simulink model "Three_Phase_Compensated_Network"  (R2021a)
settings: Solver=FixedStepDiscrete  StartTime=0.0  StopTime=0.2  FixedStep=Ts  RelTol=1e-4  EnableMultiTasking=on
PreLoadFcn:
  | Ts=50e-6;
InitFcn:
  | Ts=50e-6;
undefined symbols (not defined in the file or in its folder): D1, Delta, DiscIntNeverNeededParam
libraries: spsSeriesRLCBranchLib x6, spsBreakerLib x6, spsCurrentMeasurementLib x6, spsSurgeArresterLib x6, spsParallelRLCBranchLib x6, spsVoltageMeasurementLib x6, spsThreePhaseSeriesRLCLoadLib x4, spsLoadFlowBusLib x4, spsThreePhaseVIMeasurementLib x3, spsThreePhaseBreakerLib x2, spsDistributedParametersLineLib x2, spsThreePhaseSourceLib x1
(part 1 of 2)
settings Model: ExtModeTrigMode=oneshot  ExtModeArmWhenConnect=off  ExtModeAutoUpdateStatusClock=off  Creator=The MathWorks, Inc.  LastModifiedBy=HP
settings SolverCC: AlgebraicLoopSolver=TrustRegion
settings DataIOCC: SaveFormat=Array  ReturnWorkspaceOutputs=off  SignalLoggingName=sigsOut
settings OptimizationCC: BlockReduction=off  BooleanDataType=off  ExpressionDepthLimit=2147483647  InitFltsAndDblsToZero=on  EfficientMapNaN2IntZero=off  LifeSpan=inf
settings DebuggingCC: UnderspecifiedInitializationDetection=Classic  MergeDetectMultiDrivingBlocksExec=none  CheckExecutionContextPreStartOutputMsg=on  SignalResolutionControl=TryResolveAllWithWarning  MultiTaskDSMMsg=warning  MultiTaskCondExecSysMsg=none  FcnCallInpInsideContextMsg=warning  UnconnectedInputMsg=none  UnconnectedOutputMsg=none  StateNameClashWarn=warning  SFUnexpectedBacktrackingDiag=warning  SFNoUnconditionalDefaultTransitionDiag=warning  SFExecutionAtInitializationDiag=none  SFMachineParentedDataDiag=warning  ArithmeticOperatorsInVariantConditions=warning
settings HardwareCC: ProdBitPerPointer=32  ProdBitPerSizeT=32  ProdBitPerPtrDiffT=32  ProdLargestAtomicFloat=None  ProdIntDivRoundTo=Undefined  ProdEndianess=Unspecified  ProdWordSize=32  ProdHWDeviceType=Specified  TargetUnknown=on
settings ModelReferenceCC: PropagateSignalLabelsOutOfModel=off
settings SFSimCC: SimUseLocalCustomCode=off  CustomCodeUndefinedFunction=UseInterfaceOnly
settings RTWCC: RTWUseLocalCustomCode=off
settings CodeAppCC: StateflowObjectComments=on
settings GRTTargetCC: TargetLangStandard=C89/C90 (ANSI)  CombineOutputUpdateFcns=off  GRTInterface=on
settings ConfigComp: CovMetricSettings=dw  CovSaveCumulativeToWorkspaceVar=on  CovSaveSingleToWorkspaceVar=on  CovExternalEMLEnable=off  CovSFcnEnable=off
settings SimscapeCC: SimscapeNormalizeSystem=off

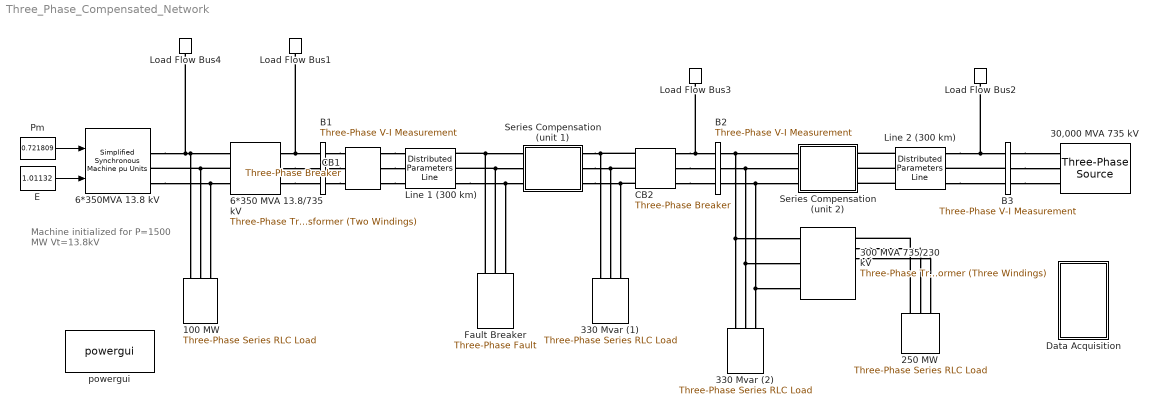
== system Three_Phase_Compensated_Network ==
  note: Machine initialized for
      |  P=1500 MW
      |  Vt=13.8kV
  100 MW : spsThreePhaseSeriesRLCLoadLib/Three-Phase Series RLC Load  LConnTagsString=A|B|C  Configuration=Y (grounded)  NominalVoltage=13.8e3  Vabc=[1e3 1e3 1e3]  Vabcp=[1e3 1e3 1e3]  NominalFrequency=60  UnbalancedPower=off  ActivePower=100000000  InductivePower=0  CapacitivePower=0  Pabc=[10e3 9e3 11e3]  QLabc=[100 90 110]  QCabc=[100 90 110]  Pabcp=[10e3 9e3 11e3]  QLabcp=[100 90 110]  QCabcp=[100 90 110]  Measurements=None  LoadType=constant Z
  250 MW : spsThreePhaseSeriesRLCLoadLib/Three-Phase Series RLC Load  LConnTagsString=A|B|C  Configuration=Y (grounded)  NominalVoltage=230e3  Vabc=[1e3 1e3 1e3]  Vabcp=[1e3 1e3 1e3]  NominalFrequency=60  UnbalancedPower=off  ActivePower=250000000  InductivePower=0  CapacitivePower=0  Pabc=[10e3 9e3 11e3]  QLabc=[100 90 110]  QCabc=[100 90 110]  Pabcp=[10e3 9e3 11e3]  QLabcp=[100 90 110]  QCabcp=[100 90 110]  Measurements=None  LoadType=constant Z
  30,000 MVA 735 kV : spsThreePhaseSourceLib/Three-Phase Source  InternalConnection=Yg  VoltagePhases=off  Voltage=(735000)*0.98865  PhaseAngle=-2.0892  Voltage_phases=[25e3 25e3 25e3]/sqrt(3)  PhaseAngles_phases=[0 -120 +120]  Frequency=60  NonIdealSource=on  SpecifyImpedance=on  Resistance=735^2/30000/10  Inductance=735^2/30000/377  ShortCircuitLevel=30000e6  BaseVoltage=735e3  XRratio=10  BusType=swing  Pref=0  Qref=0  Prefabc=[10e3, 10e3, 10e3]  Qrefabc=[0, 0, 0]  Qmin=-Inf  Qmax=Inf
  300 MVA 735/230 kV : spsThreePhaseTransformerThreeWindingsLib/Three-Phase Transformer (Three Windings)  Winding1Connection=Yg  Winding2Connection=Yg  Winding3Connection=Delta (D1)  CoreType=Three single-phase transformers  SetSaturation=on  Hysteresis=off  DataFile='hysteresis'  SetInitialFlux=off  Measurements=None  UNITS=pu  NominalPower=[ 300e6 , 60 ]  Winding1=[ 735e3 , 0.002 , 0.15 ]  Winding2=[ 230e3 , 0.002 , 0 ]  Winding3=[ 25e3 , 0.05 , 0.20 ]  Rm=500  Lm=1000  L0=0.5  Saturation="[  0,0  ;  0.0012,1.2  ;  1.0,1.45 ]"  InitialFluxes=[-1.02015948080927 0.506449133666723 0.513710347142544]  BreakLoop=on  DiscreteSolver=Trapezoidal iterative  DataType=off  TransfoNumber=0
      settings: AttributesFormatString=\n  SourceProductBaseCode=PS
  330 Mvar (1) : spsThreePhaseSeriesRLCLoadLib/Three-Phase Series RLC Load  LConnTagsString=A|B|C  Configuration=Y (grounded)  NominalVoltage=735e3  Vabc=[1e3 1e3 1e3]  Vabcp=[1e3 1e3 1e3]  NominalFrequency=60  UnbalancedPower=off  ActivePower=1320000  InductivePower=330e6  CapacitivePower=0  Pabc=[10e3 9e3 11e3]  QLabc=[100 90 110]  QCabc=[100 90 110]  Pabcp=[10e3 9e3 11e3]  QLabcp=[100 90 110]  QCabcp=[100 90 110]  Measurements=None  LoadType=constant Z
  "330 Mvar (2) " : spsThreePhaseSeriesRLCLoadLib/Three-Phase Series RLC Load  LConnTagsString=A|B|C  Configuration=Y (grounded)  NominalVoltage=735e3  Vabc=[1e3 1e3 1e3]  Vabcp=[1e3 1e3 1e3]  NominalFrequency=60  UnbalancedPower=off  ActivePower=1320000  InductivePower=330e6  CapacitivePower=0  Pabc=[10e3 9e3 11e3]  QLabc=[100 90 110]  QCabc=[100 90 110]  Pabcp=[10e3 9e3 11e3]  QLabcp=[100 90 110]  QCabcp=[100 90 110]  Measurements=None  LoadType=constant Z
  6*350 MVA 13.8/735 kV : spsThreePhaseTransformerTwoWindingsLib/Three-Phase Transformer (Two Windings)  Winding1Connection=Delta (D1)  Winding2Connection=Yg  CoreType=Three single-phase transformers  SetSaturation=off  Hysteresis=off  DataFile='hysteresis'  SetInitialFlux=off  Measurements=None  UNITS=pu  NominalPower=[ 6*350e6 , 60 ]  Winding1=[ 13.8e3 , 0.002 , 0.08 ]  Winding2=[ 735e3 , 0.002 , 0.08 ]  Rm=500  Lm=500  L0=0.5  Saturation=[ 0,0 ; 0.0024,1.2 ; 1.0,1.52 ]  InitialFluxes=[ 0.8 , -0.8 , 0.7 ]  BreakLoop=off  DiscreteSolver=Trapezoidal iterative  DataType=off  TransfoNumber=0
  6*350MVA 13.8 kV : spsSimplifiedSynchronousMachinepuUnitsLib/Simplified Synchronous Machine pu Units  ConnectionType=3-wire Y  MechanicalLoad=Mechanical power Pm  MeasurementBus=off  NominalParameters="[ 6*350e6 13.8e3  60 ]"  Mechanical=[ inf,0,2 ]  InternalRL="[ 0.22/15  0.22 ]"  InitialConditions=[0 1.43122 0.716215 0.716215 0.716215 -3.34575 -123.346 116.654 ]  IterativeDiscreteModel=Trapezoidal non iterative  TsBlock=-1  TsPowergui=0  LoadFlowParameters=[1,0,0,0,0]  Units=0  BusType=PV  Pref=1500000000  Qref=0  Qmin=-Inf  Qmax=Inf  PLF=0  QLF=0
      settings: AttributesFormatString=\n  SourceProductBaseCode=PS
  B1 : spsThreePhaseVIMeasurementLib/Three-Phase V-I Measurement  VoltageMeasurement=phase-to-ground  SetLabelV=on  LabelV=Vabc_B1  Vpu=on  VpuLL=off  CurrentMeasurement=yes  SetLabelI=on  LabelI=Iabc_B1  Ipu=on  Pbase=100e6  Vbase=735e3  OutputType=Complex  PhasorSimulation=off  PSBequivalent=0
  B2 : spsThreePhaseVIMeasurementLib/Three-Phase V-I Measurement  VoltageMeasurement=phase-to-ground  SetLabelV=on  LabelV=Vabc_B2  Vpu=on  VpuLL=off  CurrentMeasurement=yes  SetLabelI=on  LabelI=Iabc_B2  Ipu=on  Pbase=100e6  Vbase=735e3  OutputType=Complex  PhasorSimulation=off  PSBequivalent=0
  B3 : spsThreePhaseVIMeasurementLib/Three-Phase V-I Measurement  VoltageMeasurement=no  SetLabelV=on  LabelV=Vabc_B3  Vpu=on  VpuLL=off  CurrentMeasurement=no  SetLabelI=on  LabelI=Iabc_B3  Ipu=on  Pbase=100e6  Vbase=735e3  OutputType=Complex  PhasorSimulation=off  PSBequivalent=0
  CB1 : spsThreePhaseBreakerLib/Three-Phase Breaker  InitialState=closed  SwitchA=on  SwitchB=on  SwitchC=on  SwitchTimes="[5/60  ]"  External=off  BreakerResistance=0.001  SnubberResistance=1e5  SnubberCapacitance=inf  Measurements=None
      settings: AttributesFormatString=\n
  CB2 : spsThreePhaseBreakerLib/Three-Phase Breaker  InitialState=closed  SwitchA=on  SwitchB=on  SwitchC=on  SwitchTimes="[5/60  ]"  External=off  BreakerResistance=0.001  SnubberResistance=1e5  SnubberCapacitance=inf  Measurements=None
      settings: AttributesFormatString=\n
  Data Acquisition : Subsystem  mask(Data Acquisition){}
      mask Display: disp('Scopes')
  E : Constant  Value=1.01132
  Fault Breaker : spsThreePhaseFaultLib/Three-Phase Fault  InitialStates=0  FaultA=on  FaultB=off  FaultC=off  GroundFault=on  SwitchTimes=[ 1/60 6/60]  External=off  SwitchStatus=NaN  FaultResistance=0.001  GroundResistance=1  SnubberResistance=inf  SnubberCapacitance=inf  Measurements=Fault currents
  Line 1 (300 km) : spsDistributedParametersLineLib/Distributed Parameters Line  Phases=3  Length=300  Frequency=60  Resistance=[0.01273 0.3864]  Inductance="[0.9337e-3  4.1264e-3]"  Capacitance=[12.74e-9 7.751e-9]  x1=[-0.0017 -7.353032972499e-08 0 0;-0.00165 -7.42667095508993e-08 0 0;-0.0016 -7.49767027685348e-08 0 0;-0.00155 -7.56600571206871e-08 0 0;-0.0015 -7.63165298148087e-08 0 0;-0.00145 -7.69458876092773e-08 0 0;-0.0014 -7.75479068962652e-08 0 0;-0.00135 -7.81223737811864e-08 0 0;-0.0013 -7.86690841586921e-08 0 0;-0.00125 -7.91878437851883e-08 0 0;-0.0012 -7.96784683478498e-08 0 0;-0.00115 -8.01407835301058e-08 0 0;-0.0011 -8.05746250735734e-08 0 0;-0.00105 -8.09798388364179e-08 298982.56569214 -680729.342896262;-0.001 -8.13562808481189e-08 311760.155284904 -674973.083751637;-0.00095 -8.17038173606221e-08 324426.977978977 -668977.009884319;-0.0009 -8.20223248958594e-08 336978.533312573 -662743.251670802;-0.00085 -8.23116902896202e-08 349410.361777845 -656274.023935697;-0.0008 -8.25718107317579e-08 361718.046405336 -649571.625164814;-0.00075 -8.28025938027181e-08 373897.214333303 -642638.436688521;-0.0007 -8.30039575063745e-08 385943.538361373 -635476.921835672;-0.00065 -8.3175830299162e-08 397852.738487979 -628089.625058393;-0.0006 -8.33181511154957e-08 409620.583431022 -620479.171028054;-0.00055 -8.34308693894673e-08 421242.89213123 -612648.263702733;-0.0005 -8.35139450728108e-08 432715.535237661 -604599.685366516;-0.00045 -8.35673486491314e-08 444034.436574848 -596336.29564096;-0.0004 -8.35910611443928e-08 455195.574591042 -587861.030469089;-0.00035 -8.35850741336582e-08 466194.983787052 -579176.901072262;-0.0003 -8.35493897440842e-08 477028.756125164 -570286.992880304;-0.00025 -8.34840206541644e-08 487693.042417654 -561194.464435263;-0.0002 -8.33889900892251e-08 498184.053694381 -551902.546269203;-0.00015 -8.32643318131737e-08 508498.062548993 -542414.539756402;-0.0001 -8.3110090116502e-08 518631.404463254 -532733.815940397;-5e-05 -8.29263198005504e-08 528580.479109035 -522863.814336262]  x2=[-0.0017 -2.16943566485558e-08 0 0;-0.00165 -2.19441858844851e-08 0 0;-0.0016 -2.21862184556595e-08 0 0;-0.00155 -2.24203683690588e-08 0 0;-0.0015 -2.26465524323339e-08 0 0;-0.00145 -2.2864690283364e-08 0 0;-0.0014 -2.30747044188093e-08 0 0;-0.00135 -2.32765202216475e-08 0 0;-0.0013 -2.34700659876849e-08 0 0;-0.00125 -2.36552729510324e-08 0 0;-0.0012 -2.38320753085377e-08 0 0;-0.00115 -2.40004102431651e-08 0 0;-0.0011 -2.4160217946314e-08 0 0;-0.00105 -2.43114416390682e-08 112715.55611075 -734159.055210883;-0.001 -2.44540275923699e-08 126533.2909278 -731904.127817148;-0.00095 -2.45879251461087e-08 140306.069069085 -729389.158371848;-0.0009 -2.47130867271215e-08 154028.997132115 -726615.040431651;-0.00085 -2.48294678660944e-08 167697.199425891 -723582.759627452;-0.0008 -2.49370272133628e-08 181305.81970322 -720293.393314182;-0.00075 -2.5035726553603e-08 194850.022886119 -716748.11018803;-0.0007 -2.51255308194093e-08 208324.996783687 -712948.169871208;-0.00065 -2.52064081037536e-08 221725.953801862 -708894.922464418;-0.0006 -2.52783296713219e-08 235048.132644425 -704589.808067163;-0.00055 -2.53412699687238e-08 248286.80000467 -700034.35626609;-0.0005 -2.53952066335712e-08 261437.252247119 -695230.185591531;-0.00045 -2.54401205024239e-08 274494.81707871 -690179.002942453;-0.0004 -2.54759956175983e-08 287454.855208832 -684882.602979997;-0.00035 -2.55028192328368e-08 300312.761997648 -679342.867489852;-0.0003 -2.55205818178365e-08 313063.969092102 -673561.76471366;-0.00025 -2.55292770616355e-08 325703.946049028 -667541.348649708;-0.0002 -2.55289018748553e-08 338228.2019448 -661283.758323158;-0.00015 -2.55194563907977e-08 350632.286970935 -654791.217026056;-0.0001 -2.55009439653985e-08 362911.794015086 -648066.031527411;-5e-05 -2.54733711760341e-08 375062.360226872 -641110.591253607]  x3=[-0.0017 -1.01423419492597e-10 0 0;-0.00165 -1.00706128675162e-10 0 0;-0.0016 -9.9953057449734e-11 0 0;-0.00155 -9.9164473378932e-11 0 0;-0.0015 -9.83406566429218e-11 0 0;-0.00145 -9.7481899939867e-11 0 0;-0.0014 -9.65885083819351e-11 0 0;-0.00135 -9.56607993868927e-11 0 0;-0.0013 -9.46991025653284e-11 0 0;-0.00125 -9.37037596035435e-11 0 0;-0.0012 -9.2675124142153e-11 0 0;-0.00115 -9.16135616504384e-11 0 0;-0.0011 -9.05194492964981e-11 0 0;-0.00105 -8.93931758132418e-11 21.8468552412291 -927.931576584709;-0.001 -8.82351413602752e-11 39.332930122682 -927.355137167526;-0.00095 -8.70457573817254e-11 56.8050302013506 -926.449212885817;-0.0009 -8.58254464600565e-11 74.2569477232727 -925.214125610167;-0.00085 -8.45746421659283e-11 91.6824821052518 -923.650314161204;-0.0008 -8.32937889041507e-11 109.075442137896 -921.75833415369;-0.00075 -8.19833417557887e-11 126.429648185324 -919.538857799112;-0.0007 -8.06437663164742e-11 143.738934380762 -916.992673666851;-0.00065 -7.92755385309822e-11 160.997150817243 -914.120686404005;-0.0006 -7.78791445241301e-11 178.198165732647 -910.923916413973;-0.00055 -7.64550804280592e-11 195.335867688277 -907.403499493911;-0.0005 -7.50038522059622e-11 212.404167740233 -903.560686431188;-0.00045 -7.3525975472316e-11 229.397001602778 -899.396842558986;-0.0004 -7.20219753096872e-11 246.308331802954 -894.913447271207;-0.00035 -7.0492386082172e-11 263.132149825667 -890.112093496849;-0.0003 -6.89377512455396e-11 279.862478248481 -884.994487134046;-0.00025 -6.73586231541448e-11 296.493372865373 -879.562446443969;-0.0002 -6.57555628646795e-11 313.018924798673 -873.817901404811;-0.00015 -6.41291399368312e-11 329.433262598469 -867.762893026071;-0.0001 -6.24799322309218e-11 345.730554328699 -861.399572623394;-5e-05 -6.08085257025963e-11 361.905009639212 -854.73020105422]  x4=[-0.0017 8.61697744654709e-12 0 0;-0.00165 5.94163974360045e-12 0 0;-0.0016 3.26419100434471e-12 0 0;-0.00155 5.85582513567954e-13 0 0;-0.0015 -2.09323403188755e-12 0 0;-0.00145 -4.77130686125871e-12 0 0;-0.0014 -7.44768446802119e-12 0 0;-0.00135 -1.01214159479552e-11 0 0;-0.0013 -1.27915513369973e-11 0 0;-0.00125 -1.54571419487578e-11 0 0;-0.0012 -1.81172407115849e-11 0 0;-0.00115 -2.07709025050545e-11 0 0;-0.0011 -2.34171844957672e-11 0 0;-0.00105 -2.60551464723323e-11 457.510949143643 -4541.09394571612;-0.001 -2.86838511794203e-11 543.022422494244 -4531.66378032676;-0.00095 -3.13023646507659e-11 628.340962563797 -4520.62353637429;-0.0009 -3.3909756541001e-11 713.436256081272 -4507.97713640484;-0.00085 -3.65051004562023e-11 798.278069094071 -4493.72907362409;-0.0008 -3.9087474283035e-11 882.836257710017 -4477.88441030089;-0.00075 -4.16559605163744e-11 967.080778807328 -4460.4487759687;-0.0007 -4.42096465852922e-11 1050.9817007088 -4441.42836542535;-0.00065 -4.67476251772877e-11 1134.50921381638 -4420.82993653216;-0.0006 -4.9268994560652e-11 1217.63364120239 -4398.66080781282;-0.00055 -5.1772858904849e-11 1300.32544915359 -4374.9288558532;-0.0005 -5.42583285987998e-11 1382.55525766436 -4349.64251250284;-0.00045 -5.67245205669568e-11 1464.29385087528 -4322.81076187913;-0.0004 -5.91705585830569e-11 1545.51218745339 -4294.44313717529;-0.00035 -6.159557358144e-11 1626.18141091044 -4264.54971727331;-0.0003 -6.39987039658242e-11 1706.27285985544 -4233.14112316294;-0.00025 -6.63790959154267e-11 1785.75807817796 -4200.22851416812;-0.0002 -6.87359036883224e-11 1864.6088251584 -4165.82358398209;-0.00015 -7.10682899219318e-11 1942.79708550182 -4129.93855651273;-0.0001 -7.33754259305319e-11 2020.29507929161 -4092.58618153944;-5e-05 -7.56564919996847e-11 2097.07527185961 -4053.77973018318]  x5=0.00169662470098723  V1=ones(3,3)  V2=ones(3,3)  I1=ones(3,3)  I2=ones(3,3)  nHarmo=1  Measurements=None  Decoupling=off  VsMag0=0  VrMag0=0  VsAngle0=0  VrAngle0=0  IsMag0=0  IrMag0=0  IsAngle0=0  IrAngle0=0
      settings: AttributesFormatString=\n  SourceProductBaseCode=PS
  Line 2 (300 km) : spsDistributedParametersLineLib/Distributed Parameters Line  Phases=3  Length=300  Frequency=60  Resistance=[0.01273 0.3864]  Inductance="[0.9337e-3  4.1264e-3]"  Capacitance=[12.74e-9 7.751e-9]  x1=[-0.0017 -2.9133970757706e-08 0 0;-0.00165 -2.9387158290839e-08 0 0;-0.0016 -2.96299047065616e-08 0 0;-0.00155 -2.98621237582283e-08 0 0;-0.0015 -3.00837329395157e-08 0 0;-0.00145 -3.02946535137369e-08 0 0;-0.0014 -3.04948105418163e-08 0 0;-0.00135 -3.06841329089148e-08 0 0;-0.0013 -3.08625533496969e-08 0 0;-0.00125 -3.10300084722295e-08 0 0;-0.0012 -3.1186438780505e-08 0 0;-0.00115 -3.13317886955797e-08 0 0;-0.0011 -3.14660065753209e-08 0 0;-0.00105 -3.1589044732755e-08 246177.226114308 -694466.011958518;-0.001 -3.17008594530104e-08 259223.108712888 -689702.607076716;-0.00095 -3.18014110088496e-08 272176.890575264 -684694.154142719;-0.0009 -3.18906636747836e-08 285033.969284421 -679442.432636007;-0.00085 -3.1968585739765e-08 297789.776781514 -673949.308468226;-0.0008 -3.20351495184553e-08 310439.780988878 -668216.733320234;-0.00075 -3.20903313610608e-08 322979.487420252 -662246.743948687;-0.0007 -3.21341116617357e-08 335404.44077765 -656041.461462381;-0.00065 -3.21664748655475e-08 347710.226534308 -649603.090568636;-0.0006 -3.2187409474004e-08 359892.472503142 -642933.918789974;-0.00055 -3.21969080491386e-08 371946.850390165 -636036.315651371;-0.0005 -3.21949672161527e-08 383869.077332315 -628912.73183838;-0.00045 -3.2181587664615e-08 395654.917419125 -621565.698326408;-0.0004 -3.21567741482165e-08 407300.183197734 -613997.82548148;-0.00035 -3.21205354830815e-08 418800.737160661 -606211.802132781;-0.0003 -3.2072884544635e-08 430152.493215844 -598210.394617333;-0.00025 -3.20138382630286e-08 441351.41813841 -589996.445797128;-0.0002 -3.1943417617125e-08 452393.533003657 -581572.874049068;-0.00015 -3.18616476270445e-08 463274.914600754 -572942.672228086;-0.0001 -3.1768557345275e-08 473991.696826631 -564108.906603796;-5e-05 -3.16641798463505e-08 484540.072059593 -555074.715771061]  x2=[-0.0017 -1.49705866123656e-09 0 0;-0.00165 -1.5048376323934e-09 0 0;-0.0016 -1.5120819419049e-09 0 0;-0.00155 -1.5187890159024e-09 0 0;-0.0015 -1.52495647139445e-09 0 0;-0.00145 -1.53058211711347e-09 0 0;-0.0014 -1.53566395429432e-09 0 0;-0.00135 -1.54020017738446e-09 0 0;-0.0013 -1.54418917468542e-09 0 0;-0.00125 -1.54762952892546e-09 0 0;-0.0012 -1.55052001776308e-09 0 0;-0.00115 -1.55285961422138e-09 0 0;-0.0011 -1.55464748705288e-09 0 0;-0.00105 -1.55588300103485e-09 93647.5489574696 -729009.852352179;-0.001 -1.55656571719509e-09 107371.613342242 -727115.238496599;-0.00095 -1.55669539296777e-09 121057.529104057 -724962.284059025;-0.0009 -1.55627198227972e-09 134700.433702212 -722551.753973919;-0.00085 -1.55529563556674e-09 148295.479877663 -719884.504691141;-0.0008 -1.55376669972017e-09 161837.837375241 -716961.483871662;-0.00075 -1.55168571796363e-09 175322.694659809 -713783.73005086;-0.0007 -1.54905342966003e-09 188745.260625784 -710352.372269536;-0.00065 -1.54587077004887e-09 202100.766299392 -706668.629672771;-0.0006 -1.54213886991397e-09 215384.46653306 -702733.81107677;-0.00055 -1.53785905518166e-09 228591.641691347 -698549.314503843;-0.0005 -1.53303284644973e-09 241717.599327808 -694116.626685698;-0.00045 -1.52766195844719e-09 254757.675852195 -689437.32253521;-0.0004 -1.52174829942495e-09 267707.238187409 -684513.064586862;-0.00035 -1.5152939704779e-09 280561.685415616 -679345.602406056;-0.0003 -1.5083012647984e-09 293316.450412922 -673936.7719675;-0.00025 -1.50077266686147e-09 305967.001472057 -668288.495002893;-0.0002 -1.49271085154211e-09 318508.843912467 -662402.778318146;-0.00015 -1.48411868316492e-09 330937.521677252 -656281.713080371;-0.0001 -1.4749992144864e-09 343248.618916384 -649927.474074902;-5e-05 -1.46535568561036e-09 355437.761555633 -643342.318932601]  x3=[-0.0017 -4.36527126784884e-11 0 0;-0.00165 -4.30284895025329e-11 0 0;-0.0016 -4.23889785091424e-11 0 0;-0.00155 -4.17344069135277e-11 0 0;-0.0015 -4.106500728186e-11 0 0;-0.00145 -4.03810174486409e-11 0 0;-0.0014 -3.96826804322012e-11 0 0;-0.00135 -3.89702443483578e-11 0 0;-0.0013 -3.82439623222588e-11 0 0;-0.00125 -3.75040923984498e-11 0 0;-0.0012 -3.67508974491919e-11 0 0;-0.00115 -3.5984645081064e-11 0 0;-0.0011 -3.52056075398839e-11 0 0;-0.00105 -3.44140616139805e-11 12.2377893957578 -1258.52081063275;-0.001 -3.36102885358524e-11 35.956653477519 -1258.06675540882;-0.00095 -3.27945738822467e-11 59.6627423315112 -1257.16571505711;-0.0009 -3.1967207472696e-11 83.3476332972445 -1255.818009713;-0.00085 -3.11284832665458e-11 107.002911245737 -1254.02411820975;-0.0008 -3.0278699258513e-11 130.62017156937 -1251.78467790849;-0.00075 -2.94181573728093e-11 154.191023168009 -1249.10048447169;-0.0007 -2.8547163355869e-11 177.707091430315 -1245.9724915805;-0.00065 -2.7666026667719e-11 201.160021209208 -1242.40181059589;-0.0006 -2.67750603720291e-11 224.541479790414 -1238.38971016382;-0.00055 -2.58745810248816e-11 247.84315985303 -1233.93761576447;-0.0005 -2.49649085623008e-11 271.056782421085 -1229.04710920577;-0.00045 -2.40463661865812e-11 294.174099805015 -1223.71992806143;-0.0004 -2.31192802514551e-11 317.186898532029 -1217.95796505354;-0.00035 -2.21839801461408e-11 340.087002264317 -1211.76326738011;-0.0003 -2.12407981783123e-11 362.866274704065 -1205.13803598774;-0.00025 -2.02900694560316e-11 385.516622484241 -1198.08462478958;-0.0002 -1.93321317686867e-11 408.029998044132 -1190.60553982906;-0.00015 -1.83673254669766e-11 430.3984024886 -1182.70343838945;-0.0001 -1.73959933419863e-11 452.613888430057 -1174.38112804976;-5e-05 -1.64184805033947e-11 474.66856281213 -1165.64156568723]  x4=[-0.0017 1.18474608216593e-11 0 0;-0.00165 1.06588891254234e-11 0 0;-0.0016 9.46653037663484e-12 0 0;-0.00155 8.27080821467944e-12 0 0;-0.0015 7.07214747394779e-12 0 0;-0.00145 5.8709740328935e-12 0 0;-0.0014 4.66771466272068e-12 0 0;-0.00135 3.46279687575406e-12 0 0;-0.0013 2.256648773546e-12 0 0;-0.00125 1.049698894774e-12 0 0;-0.0012 -1.57623937017053e-13 0 0;-0.00115 -1.36489076577383e-12 0 0;-0.0011 -2.5716726553406e-12 0 0;-0.00105 -3.77754084185826e-12 198.236296947649 -4189.81019371948;-0.001 -4.98206688610202e-12 277.172661591193 -4185.32933734591;-0.00095 -6.18482282570383e-12 356.010548107863 -4179.36145338773;-0.0009 -7.38538132720546e-12 434.721945771978 -4171.90866220568;-0.00085 -8.58331583788787e-12 513.27888879874 -4162.97361174098;-0.0008 -9.77820073732356e-12 591.653466280349 -4152.55947657453;-0.00075 -1.09696114885973e-11 669.817832102616 -4140.66995679895;-0.0007 -1.21571247891423e-11 747.744214838555 -4127.309276704;-0.00065 -1.33403187211373e-11 825.404927615433 -4112.48218327572;-0.0006 -1.45187729014122e-11 902.772377951793 -4096.19394450978;-0.00055 -1.5692068630808e-11 979.819077560924 -4078.45034753987;-0.0005 -1.6859789042939e-11 1056.51765211732 -4059.2576965815;-0.00045 -1.80215192523028e-11 1132.84085098265 -4038.62281069218;-0.0004 -1.9176846501688e-11 1208.76155688779 -4016.55302134859;-0.00035 -2.03253603088238e-11 1284.25279556742 -3993.05616984181;-0.0003 -2.14666526122236e-11 1359.28774534391 -3968.14060449129;-0.00025 -2.26003179161662e-11 1433.83974665689 -3941.81517767877;-0.0002 -2.37259534347674e-11 1507.88231153528 -3914.08924270303;-0.00015 -2.4843159235087e-11 1581.38913300834 -3884.97265045676;-0.0001 -2.59515383792241e-11 1654.33409445241 -3854.47574592654;-5e-05 -2.70506970653463e-11 1726.69127887003 -3822.60936451733]  x5=0.00169662470098723  V1=ones(3,3)  V2=ones(3,3)  I1=ones(3,3)  I2=ones(3,3)  nHarmo=1  Measurements=None  Decoupling=off  VsMag0=0  VrMag0=0  VsAngle0=0  VrAngle0=0  IsMag0=0  IrMag0=0  IsAngle0=0  IrAngle0=0
      settings: AttributesFormatString=\n  SourceProductBaseCode=PS
  Load Flow Bus1 : spsLoadFlowBusLib/Load Flow Bus  LConnTagsString=a  Phases=single  Connectors=on one side  ID=B1  Vbase=735e3  Vref=1  Vangle=0  VLF=1.012  VLFb=1  VLFc=1  angleLF=16.39  angleLFb=0  angleLFc=0
      settings: AttributesFormatString=%<ID>\n%<Vbase>V\n%<VLF>pu\n%<angleLF>deg.  SourceProductBaseCode=PS
  Load Flow Bus2 : spsLoadFlowBusLib/Load Flow Bus  LConnTagsString=a  Phases=single  Connectors=on one side  ID=B3  Vbase=735e3  Vref=1  Vangle=0  VLF=1  VLFb=1  VLFc=1  angleLF=0  angleLFb=0  angleLFc=0
      settings: AttributesFormatString=%<ID>\n%<Vbase>V\n%<VLF>pu\n%<angleLF>deg.  SourceProductBaseCode=PS
  Load Flow Bus3 : spsLoadFlowBusLib/Load Flow Bus  LConnTagsString=a  Phases=single  Connectors=on one side  ID=B2  Vbase=735e3  Vref=1  Vangle=0  VLF=1.03  VLFb=1  VLFc=1  angleLF=7.354  angleLFb=0  angleLFc=0
      settings: AttributesFormatString=%<ID>\n%<Vbase>V\n%<VLF>pu\n%<angleLF>deg.  SourceProductBaseCode=PS
  Load Flow Bus4 : spsLoadFlowBusLib/Load Flow Bus  LConnTagsString=a  Phases=single  Connectors=on one side  ID=GEN  Vbase=13.8e3  Vref=1  Vangle=0  VLF=1  VLFb=1  VLFc=1  angleLF=-7.552  angleLFb=0  angleLFc=0
      settings: AttributesFormatString=%<ID>\n%<Vbase>V\n%<VLF>pu\n%<angleLF>deg.  SourceProductBaseCode=PS
  Pm : Constant  Value=0.721809
  "Series Compensation (unit 1) " : Subsystem
      mask Display: plot(0,0,100,100,[25 45],[50 50], [45 45],[35 65],[55 55],[35 65], [55 75],[50 50])
  "Series Compensation (unit 2) " : Subsystem
      mask Display: plot(0,0,100,100,[25 45],[50 50], [45 45],[35 65],[55 55],[35 65], [55 75],[50 50])
  powergui : spspowerguiLib/powergui  Priority=2  SimulationMode=Discrete  SampleTime=Ts  frequency=60  Iterations=50  frequencyindice=60  Pbase=100e6  ErrMax=0.0001  UnitsV=kV  UnitsW=MW  buscounter=0  FunctionMessages=off  echomessages=off  EnableUseOfTLC=off  CurrentSourceSwitches=off  DisableSnubberDevices=off  DisableRonSwitches=off  DisableVfSwitches=off  DisplayEquations=off  AutomaticDiscreteSolvers=off  SolverType=Tustin/Backward Euler (TBE)  Interpol=off  ExternalGateDelay=off  methode=off  Ts=0  x0status=blocks  SPID=off  SwTol=0  HookPort=off  NonlinearTolerance=1e-4  nMaxIteration=100  ContinueOnMaxIteration=off  RestoreLinks=warning  ResistiveCurrentMeasurement=off  Frange=0:0.5:500  Ylog=off  Xlog=off  ShowGrid=off  save=on  variable=Zmes  structure=0  ZoomFFT=on  StartTime=0.0  cycles=1  DisplayStyle=off  fundamental=60  FreqAxis=off  MaxFrequency=1000  frequencyindicesteady=1  RmsSteady=1  display=off
  wires:
  Pm/1 -> 6*350MVA 13.8 kV/1
  E/1 -> 6*350MVA 13.8 kV/2
  connections:
  6*350 MVA 13.8/735 kV/LConn2 -- 6*350MVA 13.8 kV/RConn2 -- 100 MW/LConn2
  6*350MVA 13.8 kV/RConn1 -- 6*350 MVA 13.8/735 kV/LConn1 -- 100 MW/LConn1 -- Load Flow Bus4/LConn1
  6*350MVA 13.8 kV/RConn3 -- 6*350 MVA 13.8/735 kV/LConn3 -- 100 MW/LConn3
  6*350 MVA 13.8/735 kV/RConn2 -- B1/LConn2
  6*350 MVA 13.8/735 kV/RConn1 -- B1/LConn1 -- Load Flow Bus1/LConn1
  6*350 MVA 13.8/735 kV/RConn3 -- B1/LConn3
  B1/RConn2 -- CB1/LConn2
  B1/RConn1 -- CB1/LConn1
  B1/RConn3 -- CB1/LConn3
  CB1/RConn2 -- Line 1 (300 km)/LConn2
  CB1/RConn1 -- Line 1 (300 km)/LConn1
  CB1/RConn3 -- Line 1 (300 km)/LConn3
  Fault Breaker/LConn2 -- Line 1 (300 km)/RConn2 -- "Series Compensation (unit 1) "/LConn2
  Fault Breaker/LConn1 -- Line 1 (300 km)/RConn1 -- "Series Compensation (unit 1) "/LConn1
  Line 1 (300 km)/RConn3 -- Fault Breaker/LConn3 -- "Series Compensation (unit 1) "/LConn3
  CB2/RConn2 -- B2/LConn2
  CB2/RConn1 -- B2/LConn1 -- Load Flow Bus3/LConn1
  CB2/RConn3 -- B2/LConn3
  CB2/LConn2 -- 330 Mvar (1)/LConn2 -- "Series Compensation (unit 1) "/RConn2
  CB2/LConn3 -- 330 Mvar (1)/LConn3 -- "Series Compensation (unit 1) "/RConn3
  CB2/LConn1 -- 330 Mvar (1)/LConn1 -- "Series Compensation (unit 1) "/RConn1
  B2/RConn2 -- "330 Mvar (2) "/LConn2 -- 300 MVA 735/230 kV/LConn2 -- "Series Compensation (unit 2) "/LConn2
  B2/RConn3 -- "330 Mvar (2) "/LConn3 -- 300 MVA 735/230 kV/LConn3 -- "Series Compensation (unit 2) "/LConn3
  B2/RConn1 -- "330 Mvar (2) "/LConn1 -- 300 MVA 735/230 kV/LConn1 -- "Series Compensation (unit 2) "/LConn1
  300 MVA 735/230 kV/RConn2 -- 250 MW/LConn2
  250 MW/LConn1 -- 300 MVA 735/230 kV/RConn1
  300 MVA 735/230 kV/RConn3 -- 250 MW/LConn3
  Line 2 (300 km)/RConn1 -- B3/LConn1 -- Load Flow Bus2/LConn1
  B3/LConn2 -- Line 2 (300 km)/RConn2
  Line 2 (300 km)/RConn3 -- B3/LConn3
  B3/RConn3 -- 30,000 MVA 735 kV/RConn3
  B3/RConn2 -- 30,000 MVA 735 kV/RConn2
  B3/RConn1 -- 30,000 MVA 735 kV/RConn1
  Line 2 (300 km)/LConn2 -- "Series Compensation (unit 2) "/RConn2
  Line 2 (300 km)/LConn1 -- "Series Compensation (unit 2) "/RConn1
  Line 2 (300 km)/LConn3 -- "Series Compensation (unit 2) "/RConn3

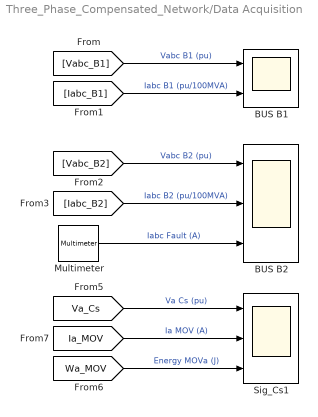
== system Three_Phase_Compensated_Network/Data Acquisition ==
  BUS B1 : Scope  NumInputPorts=2
  BUS B2 : Scope  NumInputPorts=3
  Multimeter : spsMultimeterLib/Multimeter  Tag=PoWeRsYsTeMmEaSuReMeNt  PhasorSimulation=off  OutputType=Magnitude  sel=1  L=3  Gain=1  yselected={'Ib: Fault Breaker/Fault A'};  PSBOutputType=1  PSBequivalent=0  AxesSetting=[0,0.1,-100,100]  Display=0  SavedBlockNames={}
      settings: AttributesFormatString=\n
  Sig_Cs1 : Scope  NumInputPorts=3
  wires:
  [Vabc_B1] -> BUS B1/1  "Vabc B1 (pu)"
  [Iabc_B1] -> BUS B1/2  "Iabc B1 (pu/100MVA)"
  [Vabc_B2] -> BUS B2/1  "Vabc B2 (pu)"
  [Iabc_B2] -> BUS B2/2  "Iabc B2 (pu/100MVA)"
  [Va_Cs] -> Sig_Cs1/1  "Va Cs (pu)"
  [Ia_MOV] -> Sig_Cs1/2  "Ia MOV (A)"
  [Wa_MOV] -> Sig_Cs1/3  "Energy MOVa (J)"
  Multimeter/1 -> BUS B2/3  "Iabc Fault (A)"

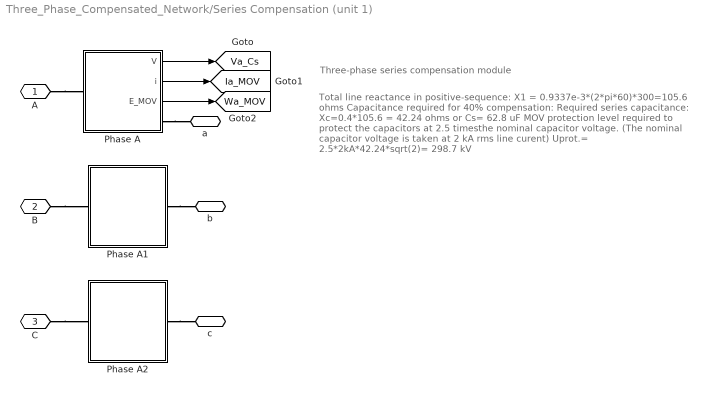
== system Three_Phase_Compensated_Network/Series Compensation (unit 1)  ==
  note: Three-phase series compensation module
  note: Total line reactance in positive-sequence:
      |  X1 = 0.9337e-3*(2*pi*60)*300=105.6 ohms
      |
      | Capacitance required for 40% compensation:
      |
      | Required series capacitance:
      | Xc=0.4*105.6 = 42.24 ohms
      | or Cs= 62.8 uF
      |
      | MOV protection level required to protect the capacitors
      | at 2.5 timesthe nominal capacitor voltage.
      | (The nominal capacitor voltage is taken at 2 kA  rms line curent)
      |
      | Uprot.= 2.5*2kA*42.24*sqrt(2)= 298.7 kV
  Phase A : Subsystem
  Phase A1 : Subsystem
  Phase A2 : Subsystem
  A : PMIOPort  Side=Left
  B : PMIOPort  Port=2  Side=Left
  C : PMIOPort  Port=3  Side=Left
  a : PMIOPort  Port=4  Side=Right
  b : PMIOPort  Port=5  Side=Right
  c : PMIOPort  Port=6  Side=Right
  tag scope: Ia_MOV=global, Va_Cs=global, Wa_MOV=global
  wires:
  Phase A/2(i) -> [Ia_MOV]
  Phase A/1(V) -> [Va_Cs]
  Phase A/3(E_MOV) -> [Wa_MOV]
  connections:
  A/RConn1 -- Phase A/LConn1
  B/RConn1 -- Phase A1/LConn1
  C/RConn1 -- Phase A2/LConn1
  Phase A/RConn1 -- a/RConn1
  Phase A1/RConn1 -- b/RConn1
  Phase A2/RConn1 -- c/RConn1

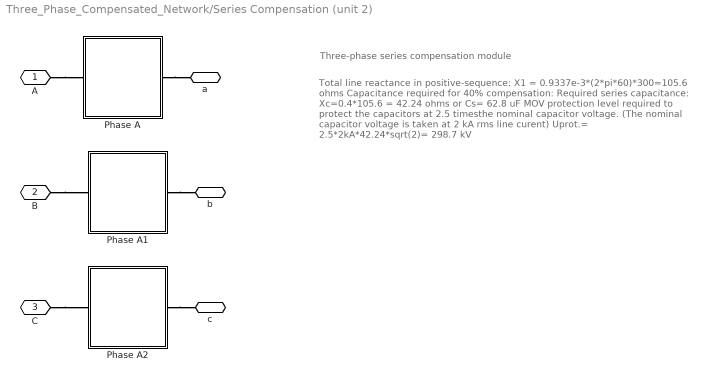
== system Three_Phase_Compensated_Network/Series Compensation (unit 2)  ==
  note: Total line reactance in positive-sequence:
      |  X1 = 0.9337e-3*(2*pi*60)*300=105.6 ohms
      |
      | Capacitance required for 40% compensation:
      |
      | Required series capacitance:
      | Xc=0.4*105.6 = 42.24 ohms
      | or Cs= 62.8 uF
      |
      | MOV protection level required to protect the capacitors
      | at 2.5 timesthe nominal capacitor voltage.
      | (The nominal capacitor voltage is taken at 2 kA  rms line curent)
      |
      | Uprot.= 2.5*2kA*42.24*sqrt(2)= 298.7 kV
  note: Three-phase series compensation module
  Phase A : Subsystem
  Phase A1 : Subsystem
  Phase A2 : Subsystem
  A : PMIOPort  Side=Left
  B : PMIOPort  Port=2  Side=Left
  C : PMIOPort  Port=3  Side=Left
  a : PMIOPort  Port=4  Side=Right
  b : PMIOPort  Port=5  Side=Right
  c : PMIOPort  Port=6  Side=Right
  connections:
  Phase A2/RConn1 -- c/RConn1
  Phase A1/RConn1 -- b/RConn1
  Phase A/RConn1 -- a/RConn1
  C/RConn1 -- Phase A2/LConn1
  B/RConn1 -- Phase A1/LConn1
  A/RConn1 -- Phase A/LConn1

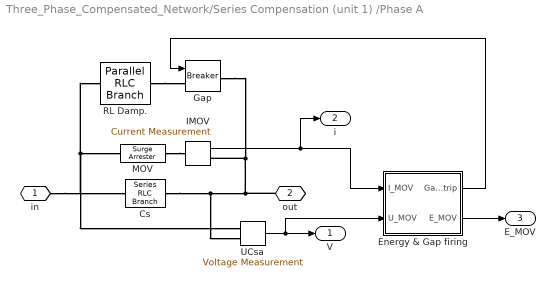
== system Three_Phase_Compensated_Network/Series Compensation (unit 1) /Phase A ==
  Cs : spsSeriesRLCBranchLib/Series RLC Branch  LConnTagsString=__new0  RConnTagsString=__new0  BranchType=C  Resistance=1.0  Inductance=1.0  SetiL0=off  InitialCurrent=0  Capacitance=62.8e-6  Setx0=off  InitialVoltage=0  Measurements=None
  Energy & Gap firing : Subsystem
  Gap : spsBreakerLib/Breaker  InitialState=0  SwitchingTimes="[ 4/60  5/60 ]"  External=on  BreakerResistance=0.001  SnubberResistance=inf  SnubberCapacitance=0  Measurements=None  MoreParameters=off  NoBreakLoop=off
      settings: AttributesFormatString=\n  SourceProductBaseCode=PS
  IMOV : spsCurrentMeasurementLib/Current Measurement  Tag=PoWeRsYsTeMmEaSuReMeNt  PhasorSimulation=off  OutputType=Magnitude  PSBequivalent=0
      settings: AttributesFormatString=\n
  MOV : spsSurgeArresterLib/Surge Arrester  ProtectionVoltage=298.7e+03  Columns=60  ReferenceCurrent=500  Segment1=[.955 50]  Segment2=[1.0 25]  Segment3=[.9915 16.5]  Measurements=None  BreakLoop=on  UseDiscreteRobustSolver=on
      settings: AttributesFormatString=\n  SourceProductBaseCode=PS
  RL Damp. : spsParallelRLCBranchLib/Parallel RLC Branch  LConnTagsString=a  RConnTagsString=__new0  BranchType=RL  Resistance=7.5  Inductance=1.7e-3  SetiL0=off  InitialCurrent=0  Capacitance=1.0  Setx0=off  InitialVoltage=0  Measurements=None
  UCsa : spsVoltageMeasurementLib/Voltage Measurement  Tag=PoWeRsYsTeMmEaSuReMeNt  PhasorSimulation=off  OutputType=Magnitude  PSBequivalent=0
  in : PMIOPort  Side=Left
  "out " : PMIOPort  Port=2  Side=Right
  V : Outport  VectorParamsAs1DForOutWhenUnconnected=off
  i : Outport  Port=2  VectorParamsAs1DForOutWhenUnconnected=off
  E_MOV : Outport  Port=3  VectorParamsAs1DForOutWhenUnconnected=off
  wires:
  Energy & Gap firing/2(E_MOV) -> E_MOV/1
  IMOV/1 -> Energy & Gap firing/1(I_MOV), i/1
  UCsa/1 -> Energy & Gap firing/2(U_MOV), V/1
  Energy & Gap firing/1(Gap_trip) -> Gap/1
  connections:
  MOV/RConn1 -- IMOV/LConn1
  Cs/LConn1 -- UCsa/LConn1 -- in/RConn1 -- RL Damp./LConn1 -- MOV/LConn1
  RL Damp./RConn1 -- Gap/LConn1
  Cs/RConn1 -- "out "/RConn1 -- IMOV/RConn1 -- Gap/RConn1 -- UCsa/LConn2

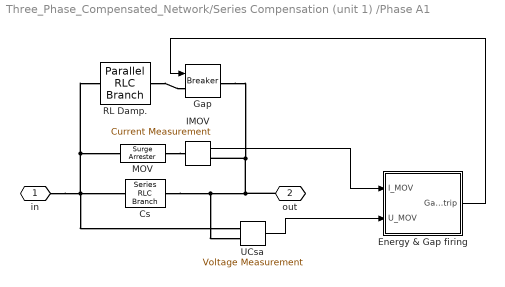
== system Three_Phase_Compensated_Network/Series Compensation (unit 1) /Phase A1 ==
  Cs : spsSeriesRLCBranchLib/Series RLC Branch  LConnTagsString=__new0  RConnTagsString=__new0  BranchType=C  Resistance=1.0  Inductance=1.0  SetiL0=off  InitialCurrent=0  Capacitance=62.8e-6  Setx0=off  InitialVoltage=0  Measurements=None
  Energy & Gap firing : Subsystem
  Gap : spsBreakerLib/Breaker  InitialState=0  SwitchingTimes="[ 4/60  5/60 ]"  External=on  BreakerResistance=0.001  SnubberResistance=inf  SnubberCapacitance=0  Measurements=None  MoreParameters=off  NoBreakLoop=off
      settings: AttributesFormatString=\n  SourceProductBaseCode=PS
  IMOV : spsCurrentMeasurementLib/Current Measurement  Tag=PoWeRsYsTeMmEaSuReMeNt  PhasorSimulation=off  OutputType=Magnitude  PSBequivalent=0
      settings: AttributesFormatString=\n
  MOV : spsSurgeArresterLib/Surge Arrester  ProtectionVoltage=298.7e+03  Columns=60  ReferenceCurrent=500  Segment1=[.955 50]  Segment2=[1.0 25]  Segment3=[.9915 16.5]  Measurements=None  BreakLoop=on  UseDiscreteRobustSolver=on
      settings: AttributesFormatString=\n  SourceProductBaseCode=PS
  RL Damp. : spsParallelRLCBranchLib/Parallel RLC Branch  LConnTagsString=a  RConnTagsString=__new0  BranchType=RL  Resistance=7.5  Inductance=1.7e-3  SetiL0=off  InitialCurrent=0  Capacitance=1.0  Setx0=off  InitialVoltage=0  Measurements=None
  UCsa : spsVoltageMeasurementLib/Voltage Measurement  Tag=PoWeRsYsTeMmEaSuReMeNt  PhasorSimulation=off  OutputType=Magnitude  PSBequivalent=0
  in : PMIOPort  Side=Left
  "out " : PMIOPort  Port=2  Side=Right
  wires:
  Energy & Gap firing/1(Gap_trip) -> Gap/1
  UCsa/1 -> Energy & Gap firing/2(U_MOV)
  IMOV/1 -> Energy & Gap firing/1(I_MOV)
  connections:
  "out "/RConn1 -- UCsa/LConn2 -- Cs/RConn1 -- Gap/RConn1 -- IMOV/RConn1
  RL Damp./RConn1 -- Gap/LConn1
  in/RConn1 -- UCsa/LConn1 -- Cs/LConn1 -- MOV/LConn1 -- RL Damp./LConn1
  MOV/RConn1 -- IMOV/LConn1

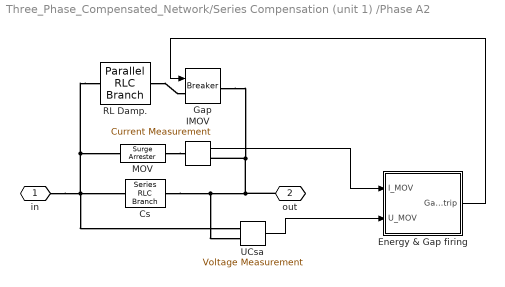
== system Three_Phase_Compensated_Network/Series Compensation (unit 1) /Phase A2 ==
  Cs : spsSeriesRLCBranchLib/Series RLC Branch  LConnTagsString=__new0  RConnTagsString=__new0  BranchType=C  Resistance=1.0  Inductance=1.0  SetiL0=off  InitialCurrent=0  Capacitance=62.8e-6  Setx0=off  InitialVoltage=0  Measurements=None
  Energy & Gap firing : Subsystem
  Gap : spsBreakerLib/Breaker  InitialState=0  SwitchingTimes="[ 4/60  5/60 ]"  External=on  BreakerResistance=0.001  SnubberResistance=inf  SnubberCapacitance=0  Measurements=None  MoreParameters=off  NoBreakLoop=off
      settings: AttributesFormatString=\n  SourceProductBaseCode=PS
  IMOV : spsCurrentMeasurementLib/Current Measurement  Tag=PoWeRsYsTeMmEaSuReMeNt  PhasorSimulation=off  OutputType=Magnitude  PSBequivalent=0
      settings: AttributesFormatString=\n
  MOV : spsSurgeArresterLib/Surge Arrester  ProtectionVoltage=298.7e+03  Columns=60  ReferenceCurrent=500  Segment1=[.955 50]  Segment2=[1.0 25]  Segment3=[.9915 16.5]  Measurements=None  BreakLoop=on  UseDiscreteRobustSolver=on
      settings: AttributesFormatString=\n  SourceProductBaseCode=PS
  RL Damp. : spsParallelRLCBranchLib/Parallel RLC Branch  LConnTagsString=a  RConnTagsString=__new0  BranchType=RL  Resistance=7.5  Inductance=1.7e-3  SetiL0=off  InitialCurrent=0  Capacitance=1.0  Setx0=off  InitialVoltage=0  Measurements=None
  UCsa : spsVoltageMeasurementLib/Voltage Measurement  Tag=PoWeRsYsTeMmEaSuReMeNt  PhasorSimulation=off  OutputType=Magnitude  PSBequivalent=0
  in : PMIOPort  Side=Left
  "out " : PMIOPort  Port=2  Side=Right
  wires:
  IMOV/1 -> Energy & Gap firing/1(I_MOV)
  UCsa/1 -> Energy & Gap firing/2(U_MOV)
  Energy & Gap firing/1(Gap_trip) -> Gap/1
  connections:
  MOV/RConn1 -- IMOV/LConn1
  RL Damp./LConn1 -- MOV/LConn1 -- Cs/LConn1 -- UCsa/LConn1 -- in/RConn1
  RL Damp./RConn1 -- Gap/LConn1
  IMOV/RConn1 -- Gap/RConn1 -- Cs/RConn1 -- UCsa/LConn2 -- "out "/RConn1

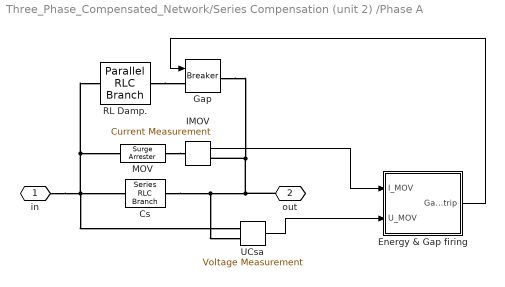
== system Three_Phase_Compensated_Network/Series Compensation (unit 2) /Phase A ==
  Cs : spsSeriesRLCBranchLib/Series RLC Branch  LConnTagsString=__new0  RConnTagsString=__new0  BranchType=C  Resistance=1.0  Inductance=1.0  SetiL0=off  InitialCurrent=0  Capacitance=62.8e-6  Setx0=off  InitialVoltage=0  Measurements=None
  Energy & Gap firing : Subsystem
  Gap : spsBreakerLib/Breaker  InitialState=0  SwitchingTimes="[ 4/60  5/60 ]"  External=on  BreakerResistance=0.001  SnubberResistance=inf  SnubberCapacitance=0  Measurements=None  MoreParameters=off  NoBreakLoop=off
      settings: AttributesFormatString=\n  SourceProductBaseCode=PS
  IMOV : spsCurrentMeasurementLib/Current Measurement  Tag=PoWeRsYsTeMmEaSuReMeNt  PhasorSimulation=off  OutputType=Magnitude  PSBequivalent=0
      settings: AttributesFormatString=\n
  MOV : spsSurgeArresterLib/Surge Arrester  ProtectionVoltage=298.7e+03  Columns=60  ReferenceCurrent=500  Segment1=[.955 50]  Segment2=[1.0 25]  Segment3=[.9915 16.5]  Measurements=None  BreakLoop=on  UseDiscreteRobustSolver=on
      settings: AttributesFormatString=\n  SourceProductBaseCode=PS
  RL Damp. : spsParallelRLCBranchLib/Parallel RLC Branch  LConnTagsString=a  RConnTagsString=__new0  BranchType=RL  Resistance=7.5  Inductance=1.7e-3  SetiL0=off  InitialCurrent=0  Capacitance=1.0  Setx0=off  InitialVoltage=0  Measurements=None
  UCsa : spsVoltageMeasurementLib/Voltage Measurement  Tag=PoWeRsYsTeMmEaSuReMeNt  PhasorSimulation=off  OutputType=Magnitude  PSBequivalent=0
  in : PMIOPort  Side=Left
  "out " : PMIOPort  Port=2  Side=Right
  wires:
  Energy & Gap firing/1(Gap_trip) -> Gap/1
  UCsa/1 -> Energy & Gap firing/2(U_MOV)
  IMOV/1 -> Energy & Gap firing/1(I_MOV)
  connections:
  "out "/RConn1 -- UCsa/LConn2 -- Cs/RConn1 -- Gap/RConn1 -- IMOV/RConn1
  RL Damp./RConn1 -- Gap/LConn1
  in/RConn1 -- UCsa/LConn1 -- Cs/LConn1 -- MOV/LConn1 -- RL Damp./LConn1
  MOV/RConn1 -- IMOV/LConn1

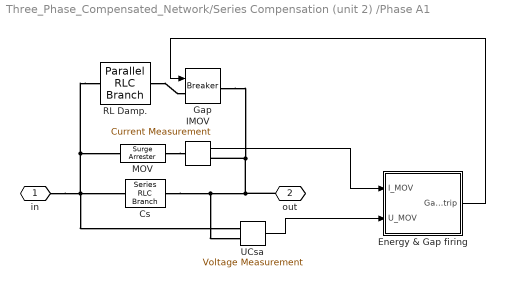
== system Three_Phase_Compensated_Network/Series Compensation (unit 2) /Phase A1 ==
  Cs : spsSeriesRLCBranchLib/Series RLC Branch  LConnTagsString=__new0  RConnTagsString=__new0  BranchType=C  Resistance=1.0  Inductance=1.0  SetiL0=off  InitialCurrent=0  Capacitance=62.8e-6  Setx0=off  InitialVoltage=0  Measurements=None
  Energy & Gap firing : Subsystem
  Gap : spsBreakerLib/Breaker  InitialState=0  SwitchingTimes="[ 4/60  5/60 ]"  External=on  BreakerResistance=0.001  SnubberResistance=inf  SnubberCapacitance=0  Measurements=None  MoreParameters=off  NoBreakLoop=off
      settings: AttributesFormatString=\n  SourceProductBaseCode=PS
  IMOV : spsCurrentMeasurementLib/Current Measurement  Tag=PoWeRsYsTeMmEaSuReMeNt  PhasorSimulation=off  OutputType=Magnitude  PSBequivalent=0
      settings: AttributesFormatString=\n
  MOV : spsSurgeArresterLib/Surge Arrester  ProtectionVoltage=298.7e+03  Columns=60  ReferenceCurrent=500  Segment1=[.955 50]  Segment2=[1.0 25]  Segment3=[.9915 16.5]  Measurements=None  BreakLoop=on  UseDiscreteRobustSolver=on
      settings: AttributesFormatString=\n  SourceProductBaseCode=PS
  RL Damp. : spsParallelRLCBranchLib/Parallel RLC Branch  LConnTagsString=a  RConnTagsString=__new0  BranchType=RL  Resistance=7.5  Inductance=1.7e-3  SetiL0=off  InitialCurrent=0  Capacitance=1.0  Setx0=off  InitialVoltage=0  Measurements=None
  UCsa : spsVoltageMeasurementLib/Voltage Measurement  Tag=PoWeRsYsTeMmEaSuReMeNt  PhasorSimulation=off  OutputType=Magnitude  PSBequivalent=0
  in : PMIOPort  Side=Left
  "out " : PMIOPort  Port=2  Side=Right
  wires:
  IMOV/1 -> Energy & Gap firing/1(I_MOV)
  UCsa/1 -> Energy & Gap firing/2(U_MOV)
  Energy & Gap firing/1(Gap_trip) -> Gap/1
  connections:
  MOV/RConn1 -- IMOV/LConn1
  RL Damp./LConn1 -- MOV/LConn1 -- Cs/LConn1 -- UCsa/LConn1 -- in/RConn1
  RL Damp./RConn1 -- Gap/LConn1
  IMOV/RConn1 -- Gap/RConn1 -- Cs/RConn1 -- UCsa/LConn2 -- "out "/RConn1

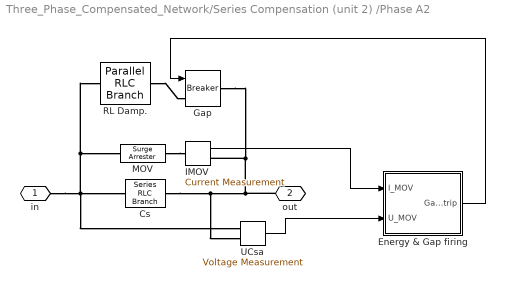
== system Three_Phase_Compensated_Network/Series Compensation (unit 2) /Phase A2 ==
  Cs : spsSeriesRLCBranchLib/Series RLC Branch  LConnTagsString=__new0  RConnTagsString=__new0  BranchType=C  Resistance=1.0  Inductance=1.0  SetiL0=off  InitialCurrent=0  Capacitance=62.8e-6  Setx0=off  InitialVoltage=0  Measurements=None
  Energy & Gap firing : Subsystem
  Gap : spsBreakerLib/Breaker  InitialState=0  SwitchingTimes="[ 4/60  5/60 ]"  External=on  BreakerResistance=0.001  SnubberResistance=inf  SnubberCapacitance=0  Measurements=None  MoreParameters=off  NoBreakLoop=off
      settings: AttributesFormatString=\n  SourceProductBaseCode=PS
  IMOV : spsCurrentMeasurementLib/Current Measurement  Tag=PoWeRsYsTeMmEaSuReMeNt  PhasorSimulation=off  OutputType=Magnitude  PSBequivalent=0
      settings: AttributesFormatString=\n
  MOV : spsSurgeArresterLib/Surge Arrester  ProtectionVoltage=298.7e+03  Columns=60  ReferenceCurrent=500  Segment1=[.955 50]  Segment2=[1.0 25]  Segment3=[.9915 16.5]  Measurements=None  BreakLoop=on  UseDiscreteRobustSolver=on
      settings: AttributesFormatString=\n  SourceProductBaseCode=PS
  RL Damp. : spsParallelRLCBranchLib/Parallel RLC Branch  LConnTagsString=a  RConnTagsString=__new0  BranchType=RL  Resistance=7.5  Inductance=1.7e-3  SetiL0=off  InitialCurrent=0  Capacitance=1.0  Setx0=off  InitialVoltage=0  Measurements=None
  UCsa : spsVoltageMeasurementLib/Voltage Measurement  Tag=PoWeRsYsTeMmEaSuReMeNt  PhasorSimulation=off  OutputType=Magnitude  PSBequivalent=0
  in : PMIOPort  Side=Left
  "out " : PMIOPort  Port=2  Side=Right
  wires:
  Energy & Gap firing/1(Gap_trip) -> Gap/1
  UCsa/1 -> Energy & Gap firing/2(U_MOV)
  IMOV/1 -> Energy & Gap firing/1(I_MOV)
  connections:
  "out "/RConn1 -- UCsa/LConn2 -- Cs/RConn1 -- Gap/RConn1 -- IMOV/RConn1
  RL Damp./RConn1 -- Gap/LConn1
  in/RConn1 -- UCsa/LConn1 -- Cs/LConn1 -- MOV/LConn1 -- RL Damp./LConn1
  MOV/RConn1 -- IMOV/LConn1

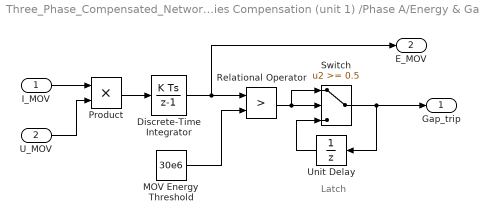
== system Three_Phase_Compensated_Network/Series Compensation (unit 1) /Phase A/Energy & Gap firing ==
  note: Latch
  I_MOV : Inport
  U_MOV : Inport  Port=2
  Discrete-Time Integrator : DiscreteIntegrator  SampleTime=Ts  ICPrevOutput=DiscIntNeverNeededParam  ICPrevScaledInput=DiscIntNeverNeededParam
  MOV Energy Threshold : Constant  Value=30e6
  Product : Product  InputSameDT=on  SaturateOnIntegerOverflow=on  OutDataTypeStr=Inherit: Same as first input
  Relational Operator : RelationalOperator  Operator=>  ZeroCross=off  RndMeth=Nearest  InputSameDT=on
  Switch : Switch  Threshold=0.5  ZeroCross=off  InputSameDT=on
  Unit Delay : UnitDelay  SampleTime=Ts  HasFrameUpgradeWarning=on
  Gap_trip : Outport  VectorParamsAs1DForOutWhenUnconnected=off
  E_MOV : Outport  Port=2  InitialOutput=0  VectorParamsAs1DForOutWhenUnconnected=off
  wires:
  Switch/1 -> Unit Delay/1, Gap_trip/1
  U_MOV/1 -> Product/2
  MOV Energy Threshold/1 -> Relational Operator/2
  Product/1 -> Discrete-Time Integrator/1
  I_MOV/1 -> Product/1
  Discrete-Time Integrator/1 -> E_MOV/1, Relational Operator/1
  Relational Operator/1 -> Switch/1, Switch/2
  Unit Delay/1 -> Switch/3

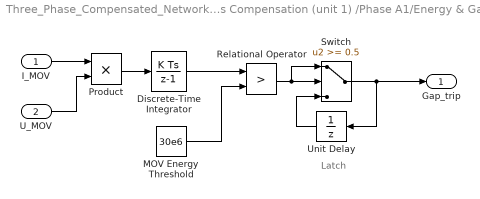
== system Three_Phase_Compensated_Network/Series Compensation (unit 1) /Phase A1/Energy & Gap firing ==
  note: Latch
  I_MOV : Inport
  U_MOV : Inport  Port=2
  Discrete-Time Integrator : DiscreteIntegrator  SampleTime=Ts  ICPrevOutput=DiscIntNeverNeededParam  ICPrevScaledInput=DiscIntNeverNeededParam
  MOV Energy Threshold : Constant  Value=30e6
  Product : Product  InputSameDT=on  SaturateOnIntegerOverflow=on  OutDataTypeStr=Inherit: Same as first input
  Relational Operator : RelationalOperator  Operator=>  ZeroCross=off  RndMeth=Nearest  InputSameDT=on
  Switch : Switch  Threshold=0.5  ZeroCross=off  InputSameDT=on
  Unit Delay : UnitDelay  SampleTime=Ts  HasFrameUpgradeWarning=on
  Gap_trip : Outport  VectorParamsAs1DForOutWhenUnconnected=off
  wires:
  Unit Delay/1 -> Switch/3
  Relational Operator/1 -> Switch/2, Switch/1
  Discrete-Time Integrator/1 -> Relational Operator/1
  I_MOV/1 -> Product/1
  Product/1 -> Discrete-Time Integrator/1
  MOV Energy Threshold/1 -> Relational Operator/2
  U_MOV/1 -> Product/2
  Switch/1 -> Gap_trip/1, Unit Delay/1

== system Three_Phase_Compensated_Network/Series Compensation (unit 1) /Phase A2/Energy & Gap firing ==
  note: Latch
  I_MOV : Inport
  U_MOV : Inport  Port=2
  Discrete-Time Integrator : DiscreteIntegrator  SampleTime=Ts  ICPrevOutput=DiscIntNeverNeededParam  ICPrevScaledInput=DiscIntNeverNeededParam
  MOV Energy Threshold : Constant  Value=30e6
  Product : Product  InputSameDT=on  SaturateOnIntegerOverflow=on  OutDataTypeStr=Inherit: Same as first input
  Relational Operator : RelationalOperator  Operator=>  ZeroCross=off  RndMeth=Nearest  InputSameDT=on
  Switch : Switch  Threshold=0.5  ZeroCross=off  InputSameDT=on
  Unit Delay : UnitDelay  SampleTime=Ts  HasFrameUpgradeWarning=on
  Gap_trip : Outport  VectorParamsAs1DForOutWhenUnconnected=off
  wires:
  Switch/1 -> Unit Delay/1, Gap_trip/1
  U_MOV/1 -> Product/2
  MOV Energy Threshold/1 -> Relational Operator/2
  Product/1 -> Discrete-Time Integrator/1
  I_MOV/1 -> Product/1
  Discrete-Time Integrator/1 -> Relational Operator/1
  Relational Operator/1 -> Switch/1, Switch/2
  Unit Delay/1 -> Switch/3

== system Three_Phase_Compensated_Network/Series Compensation (unit 2) /Phase A/Energy & Gap firing ==
  note: Latch
  I_MOV : Inport
  U_MOV : Inport  Port=2
  Discrete-Time Integrator : DiscreteIntegrator  SampleTime=Ts  ICPrevOutput=DiscIntNeverNeededParam  ICPrevScaledInput=DiscIntNeverNeededParam
  MOV Energy Threshold : Constant  Value=30e6
  Product : Product  InputSameDT=on  SaturateOnIntegerOverflow=on  OutDataTypeStr=Inherit: Same as first input
  Relational Operator : RelationalOperator  Operator=>  ZeroCross=off  RndMeth=Nearest  InputSameDT=on
  Switch : Switch  Threshold=0.5  ZeroCross=off  InputSameDT=on
  Unit Delay : UnitDelay  SampleTime=Ts  HasFrameUpgradeWarning=on
  Gap_trip : Outport  VectorParamsAs1DForOutWhenUnconnected=off
  wires:
  Unit Delay/1 -> Switch/3
  Relational Operator/1 -> Switch/2, Switch/1
  Discrete-Time Integrator/1 -> Relational Operator/1
  I_MOV/1 -> Product/1
  Product/1 -> Discrete-Time Integrator/1
  MOV Energy Threshold/1 -> Relational Operator/2
  U_MOV/1 -> Product/2
  Switch/1 -> Gap_trip/1, Unit Delay/1

== system Three_Phase_Compensated_Network/Series Compensation (unit 2) /Phase A1/Energy & Gap firing ==
  note: Latch
  I_MOV : Inport
  U_MOV : Inport  Port=2
  Discrete-Time Integrator : DiscreteIntegrator  SampleTime=Ts  ICPrevOutput=DiscIntNeverNeededParam  ICPrevScaledInput=DiscIntNeverNeededParam
  MOV Energy Threshold : Constant  Value=30e6
  Product : Product  InputSameDT=on  SaturateOnIntegerOverflow=on  OutDataTypeStr=Inherit: Same as first input
  Relational Operator : RelationalOperator  Operator=>  ZeroCross=off  RndMeth=Nearest  InputSameDT=on
  Switch : Switch  Threshold=0.5  ZeroCross=off  InputSameDT=on
  Unit Delay : UnitDelay  SampleTime=Ts  HasFrameUpgradeWarning=on
  Gap_trip : Outport  VectorParamsAs1DForOutWhenUnconnected=off
  wires:
  Switch/1 -> Unit Delay/1, Gap_trip/1
  U_MOV/1 -> Product/2
  MOV Energy Threshold/1 -> Relational Operator/2
  Product/1 -> Discrete-Time Integrator/1
  I_MOV/1 -> Product/1
  Discrete-Time Integrator/1 -> Relational Operator/1
  Relational Operator/1 -> Switch/1, Switch/2
  Unit Delay/1 -> Switch/3
